simulink model "B"  (R2013a)
settings: Solver=ode45  StartTime=0.0  StopTime=10.0  RelTol=1e-3
settings Model: Creator=Administrator  LastModifiedBy=Administrator

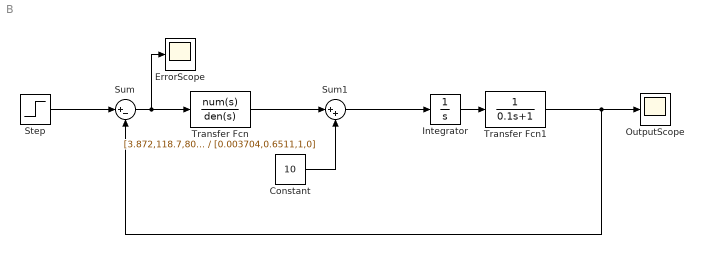
== system B ==
  Constant : Constant  Value=10
  ErrorScope : Scope
  Integrator : Integrator
  OutputScope : Scope
  Step : Step  SampleTime=0
  Sum : Sum  Inputs=|+-
  Sum1 : Sum  Inputs=|++
  Transfer Fcn : TransferFcn  Numerator=[3.872,118.7,800,0]  Denominator=[0.003704,0.6511,1,0]
  Transfer Fcn1 : TransferFcn  Denominator=[0.1 1]
  wires:
  Integrator/1 -> Transfer Fcn1/1
  Sum/1 -> Transfer Fcn/1, ErrorScope/1
  Step/1 -> Sum/1
  Transfer Fcn1/1 -> OutputScope/1, Sum/2
  Constant/1 -> Sum1/2
  Transfer Fcn/1 -> Sum1/1
  Sum1/1 -> Integrator/1
